simulink model "EcoSIM3_P2_C2_WIP"  (R2014b)
settings: Solver=ode1  SolverMode=SingleTasking  StartTime=0.0  StopTime=inf  FixedStep=0.01  RelTol=1e-3
PostLoadFcn:
  | %, if any(exist('dsrtsu_mdlpostloadfcn', 'file') == [2, 3, 6]), try dsrtsu_mdlpostloadfcn('Execute', bdroot); catch fprintf('Error in PostLoadFcn (dsrtsu_mdlpostloadfcn) for model "%s":\n %s\n', bdroot, lasterr); end, end,
InitFcn:
  | tic
  | %Startup_EcoSIM
values from neighbouring files (symbols this model uses):
  EngPwr = [0 5	10	15	20	25	30	35	40	45	50	55	60	65	70	75	80	85	90	95	100	105	110	115]    [Series_Maps.m]
  EngSpd = [0 477.4645 954.929 1909.858 2864.787 3819.716 4774.645 5729.574 6684.503]    [Series_Maps.m]
  EngTrq = [0	0	0	0	0	0	0	0	0	0	0	0	0	0	0	0	0	0	0	0	0	0	0	0 ... (first row only)    [Series_Maps.m]
  Power = [0 5 10 15 20 25 30]    [Series_Maps.m]
  Torque = [-50,-40,-30,-25,-20,-15,-10,-8,-6,-4,-2,0]    [Series_Maps.m]
undefined symbols (not defined in the file or in its folder): canChannel, Controls, DriveCycles, Driver, EM_EFF_MAP, EM_PwrLoss_MAP, Glbl, Overwritten_Mode, Plants, sigbuilder_block, Trialmap, Veh_Dynamics
libraries: simulink x141, canmsglib x113, fl_lib x104, canlib x89, nesl_utility x56, sdl_lib x29, dspsigops x6, dspswit3 x5, dspstat3 x2, commnoisgen2 x1, dspfdesign x1
(part 5 of 21)

== system EcoSIM3_P2_C2_WIP/Driver/PI Controller/Dyno Data Variant/Coastdown ==
  CycleTime : Constant  Value=Coastdown.time(end)
  From Workspace : FromWorkspace  VariableName=[Coastdown.time',Coastdown.Alpha_percent']  SampleTime=0
  From Workspace1 : FromWorkspace  VariableName=[Coastdown.time',Coastdown.Brake_percent']  SampleTime=0
  From Workspace10 : FromWorkspace  VariableName=[Coastdown.time',Coastdown.bcm_soc']  SampleTime=0
  From Workspace11 : FromWorkspace  VariableName=[Coastdown.time',Coastdown.bcm_cell_tmax']  SampleTime=0
  From Workspace12 : FromWorkspace  VariableName=[Coastdown.time',Coastdown.bcm_cell_tmin']  SampleTime=0
  From Workspace2 : FromWorkspace  VariableName=[Coastdown.time',Coastdown.Speed_m_per_s']  SampleTime=0
  From Workspace3 : FromWorkspace  VariableName=[Coastdown.time',Coastdown.Driver_Req_Trq']  SampleTime=0
  From Workspace4 : FromWorkspace  VariableName=[Coastdown.time',Coastdown.bcm_ibat']  SampleTime=0
  From Workspace5 : FromWorkspace  VariableName=[Coastdown.time',Coastdown.bcm_vbat']  SampleTime=0
  From Workspace6 : FromWorkspace  VariableName=[Coastdown.time',Coastdown.D1_Commanded_Trq']  SampleTime=0
  From Workspace7 : FromWorkspace  VariableName=[Coastdown.time',Coastdown.EM_Trq_Cmd']  SampleTime=0
  From Workspace8 : FromWorkspace  VariableName=[Coastdown.time',Coastdown.Motor_Speed']  SampleTime=0
  From Workspace9 : FromWorkspace  VariableName=[Coastdown.time',Coastdown.D2_Trq_Feedback']  SampleTime=0
  Gain : Gain
  Gain1 : Gain
  Terminator{,1..12} (13 alike) : Terminator
  n : Gain  Gain=-1
  n1 : Gain  Gain=-1
  rpmtoradps : Gain  Gain=-0.1047
  Alpha : Outport
  Beta : Outport  Port=2
  tag scope: CycleTime=global, DynoCellTMax=global, DynoCellTMin=global, DynoSpeed=global
  wires:
  Gain/1 -> Terminator8/1  "Dyno_Brk_Pct"
  From Workspace2/1 -> Terminator/1, [DynoSpeed]  "Dyno_Speed"
  From Workspace/1 -> Gain1/1, Alpha/1
  From Workspace1/1 -> Beta/1, Gain/1
  From Workspace3/1 -> Terminator1/1  "Dyno_Drv_Trq_Req"
  From Workspace5/1 -> Terminator3/1  "Dyno_bcm_vbat"
  From Workspace6/1 -> Terminator4/1  "Dyno_D1_Cmdd_Trq"
  From Workspace7/1 -> Terminator5/1  "Dyno_EM_Trq_Cmd"
  rpmtoradps/1 -> Terminator6/1  "Dyno_MotorSpd_radpers"
  From Workspace8/1 -> rpmtoradps/1  "Dyno_MotorSpd_rpm"
  n/1 -> Terminator7/1  "Dyno_D2_Trq_Fdbk"
  From Workspace9/1 -> n/1
  CycleTime/1 -> [CycleTime]
  From Workspace4/1 -> n1/1
  n1/1 -> Terminator2/1  "Dyno_bcm_ibat"
  From Workspace10/1 -> Terminator9/1  "Dyno_bcm_soc"
  Gain1/1 -> Terminator10/1  "Dyno_Alpha"
  From Workspace11/1 -> [DynoCellTMax], Terminator11/1  "Dyno_bcm_cell_tmax"
  From Workspace12/1 -> [DynoCellTMin], Terminator12/1  "Dyno_bcm_cell_tmin"

== system EcoSIM3_P2_C2_WIP/Driver/PI Controller/Dyno Data Variant/HWFET_150 ==
  CycleTime : Constant  Value=HWFET_150.time(end)
  From Workspace : FromWorkspace  VariableName=[HWFET_150.time',HWFET_150.Alpha_percent']  SampleTime=0
  From Workspace1 : FromWorkspace  VariableName=[HWFET_150.time',HWFET_150.Brake_percent']  SampleTime=0
  From Workspace10 : FromWorkspace  VariableName=[HWFET_150.time',HWFET_150.bcm_soc']  SampleTime=0
  From Workspace11 : FromWorkspace  VariableName=[HWFET_150.time',HWFET_150.bcm_cell_tmax']  SampleTime=0
  From Workspace12 : FromWorkspace  VariableName=[HWFET_150.time',HWFET_150.bcm_cell_tmin']  SampleTime=0
  From Workspace2 : FromWorkspace  VariableName=[HWFET_150.time',HWFET_150.Speed_m_per_s']  SampleTime=0
  From Workspace3 : FromWorkspace  VariableName=[HWFET_150.time',HWFET_150.Driver_Req_Trq']  SampleTime=0
  From Workspace4 : FromWorkspace  VariableName=[HWFET_150.time',HWFET_150.bcm_ibat']  SampleTime=0
  From Workspace5 : FromWorkspace  VariableName=[HWFET_150.time',HWFET_150.bcm_vbat']  SampleTime=0
  From Workspace6 : FromWorkspace  VariableName=[HWFET_150.time',HWFET_150.D1_Commanded_Trq']  SampleTime=0
  From Workspace7 : FromWorkspace  VariableName=[HWFET_150.time',HWFET_150.EM_Trq_Cmd']  SampleTime=0
  From Workspace8 : FromWorkspace  VariableName=[HWFET_150.time',HWFET_150.Motor_Speed']  SampleTime=0
  From Workspace9 : FromWorkspace  VariableName=[HWFET_150.time',HWFET_150.D2_Trq_Feedback']  SampleTime=0
  Gain : Gain
  Gain1 : Gain
  Terminator{,1..12} (13 alike) : Terminator
  Transfer Fcn : TransferFcn  Denominator=[1 1]
  n : Gain  Gain=-1
  n1 : Gain  Gain=-1
  rpmtoradps : Gain  Gain=-0.1047
  Alpha : Outport
  Beta : Outport  Port=2
  tag scope: CycleTime=global, DynoCellTMax=global, DynoCellTMin=global, DynoSpeed=global
  wires:
  Transfer Fcn/1 -> Terminator/1, [DynoSpeed]  "Dyno_Speed"
  Gain1/1 -> Terminator10/1  "Dyno_Alpha"
  From Workspace10/1 -> Terminator9/1  "Dyno_bcm_soc"
  n1/1 -> Terminator2/1  "Dyno_bcm_ibat"
  From Workspace4/1 -> n1/1
  Gain/1 -> Terminator8/1  "Dyno_Brk_Pct"
  From Workspace2/1 -> Transfer Fcn/1
  From Workspace/1 -> Alpha/1, Gain1/1
  From Workspace1/1 -> Beta/1, Gain/1
  From Workspace3/1 -> Terminator1/1  "Dyno_Drv_Trq_Req"
  From Workspace5/1 -> Terminator3/1  "Dyno_bcm_vbat"
  From Workspace6/1 -> Terminator4/1  "Dyno_D1_Cmdd_Trq"
  From Workspace7/1 -> Terminator5/1  "Dyno_EM_Trq_Cmd"
  rpmtoradps/1 -> Terminator6/1  "Dyno_MotorSpd_radpers"
  From Workspace8/1 -> rpmtoradps/1  "Dyno_MotorSpd_rpm"
  n/1 -> Terminator7/1  "Dyno_D2_Trq_Fdbk"
  From Workspace9/1 -> n/1
  CycleTime/1 -> [CycleTime]
  From Workspace11/1 -> [DynoCellTMax], Terminator11/1  "Dyno_bcm_cell_tmax"
  From Workspace12/1 -> [DynoCellTMin], Terminator12/1  "Dyno_bcm_cell_tmin"

== system EcoSIM3_P2_C2_WIP/Driver/PI Controller/Dyno Data Variant/US06_150 ==
  CycleTime : Constant  Value=US06_150.time(end)
  From Workspace : FromWorkspace  VariableName=[US06_150.time',US06_150.Alpha_percent']  SampleTime=0
  From Workspace1 : FromWorkspace  VariableName=[US06_150.time',US06_150.Brake_percent']  SampleTime=0
  From Workspace10 : FromWorkspace  VariableName=[US06_150.time',US06_150.bcm_soc']  SampleTime=0
  From Workspace11 : FromWorkspace  VariableName=[US06_150.time',US06_150.bcm_cell_tmax']  SampleTime=0
  From Workspace12 : FromWorkspace  VariableName=[US06_150.time',US06_150.bcm_cell_tmin']  SampleTime=0
  From Workspace2 : FromWorkspace  VariableName=[US06_150.time',US06_150.Speed_m_per_s']  SampleTime=0
  From Workspace3 : FromWorkspace  VariableName=[US06_150.time',US06_150.Driver_Req_Trq']  SampleTime=0
  From Workspace4 : FromWorkspace  VariableName=[US06_150.time',US06_150.bcm_ibat']  SampleTime=0
  From Workspace5 : FromWorkspace  VariableName=[US06_150.time',US06_150.bcm_vbat']  SampleTime=0
  From Workspace6 : FromWorkspace  VariableName=[US06_150.time',US06_150.D1_Commanded_Trq']  SampleTime=0
  From Workspace7 : FromWorkspace  VariableName=[US06_150.time',US06_150.EM_Trq_Cmd']  SampleTime=0
  From Workspace8 : FromWorkspace  VariableName=[US06_150.time',US06_150.Motor_Speed']  SampleTime=0
  From Workspace9 : FromWorkspace  VariableName=[US06_150.time',US06_150.D2_Trq_Feedback']  SampleTime=0
  Gain : Gain
  Gain1 : Gain
  Terminator{,1..12} (13 alike) : Terminator
  Transfer Fcn : TransferFcn  Denominator=[1 1]
  n : Gain  Gain=-1
  n1 : Gain  Gain=-1
  rpmtoradps : Gain  Gain=-0.1047
  Alpha : Outport
  Beta : Outport  Port=2
  tag scope: CycleTime=global, DynoCellTMax=global, DynoCellTMin=global, DynoSpeed=global
  wires:
  CycleTime/1 -> [CycleTime]
  From Workspace9/1 -> n/1
  n/1 -> Terminator7/1  "Dyno_D2_Trq_Fdbk"
  From Workspace8/1 -> rpmtoradps/1  "Dyno_MotorSpd_rpm"
  rpmtoradps/1 -> Terminator6/1  "Dyno_MotorSpd_radpers"
  From Workspace7/1 -> Terminator5/1  "Dyno_EM_Trq_Cmd"
  From Workspace6/1 -> Terminator4/1  "Dyno_D1_Cmdd_Trq"
  From Workspace5/1 -> Terminator3/1  "Dyno_bcm_vbat"
  From Workspace3/1 -> Terminator1/1  "Dyno_Drv_Trq_Req"
  From Workspace1/1 -> Gain/1, Beta/1
  From Workspace/1 -> Gain1/1, Alpha/1
  From Workspace2/1 -> Transfer Fcn/1
  Gain/1 -> Terminator8/1  "Dyno_Brk_Pct"
  From Workspace4/1 -> n1/1
  n1/1 -> Terminator2/1  "Dyno_bcm_ibat"
  From Workspace10/1 -> Terminator9/1  "Dyno_bcm_soc"
  Gain1/1 -> Terminator10/1  "Dyno_Alpha"
  Transfer Fcn/1 -> [DynoSpeed], Terminator/1  "Dyno_Speed"
  From Workspace11/1 -> [DynoCellTMax], Terminator11/1  "Dyno_bcm_cell_tmax"
  From Workspace12/1 -> [DynoCellTMin], Terminator12/1  "Dyno_bcm_cell_tmin"

== system EcoSIM3_P2_C2_WIP/GCM/GCM_IO/VNT Kvaser/CAN Rx ==
  note: This is a digital signal. So use from goto.
  Ground : Ground
  CAN : Outport
  wires:
  Ground/1 -> CAN/1

== system EcoSIM3_P2_C2_WIP/GCM/GCM_IO/VNT Kvaser/CAN Tx ==
  CAN : Inport
  Bus Selector : BusSelector  OutputSignals=charge_mode_request
  CAN Pack6 : canmsglib/CAN Pack  CANdbFile=C:\Users\EcoCAR_HIL\Documents\Khanna\EcoSIM3_P1_0_PHEV_TCU\Final_DBC\EcoCAR3_Controls_Development.dbc  MsgList=GCM_Transmit_MSG096  MsgName=GCM_Transmit_MSG096  MsgIDType=Standard (11-bit identifier)  MsgIdentifier=96  MsgLength=1  SignalInfo=charge_mode_request$7$1$2$2$1$0$1$0$0$1$#  NSignals=1  StartBits=str2num('[int32(7)]')  SignalSizes=str2num('[int32(1)]')  ByteOrders=str2num('[int32(2)]')  DataTypes=str2num('[int32(2)]')  MultiplexTypes=str2num('[int32(1)]')  MultiplexValues=str2num('[double(0)]')  Factors=str2num('[double(1)]')  Offsets=str2num('[double(0)]')  Minimums=str2num('[double(0)]')  Maximums=str2num('[double(1)]')  Remote=off
      settings: DataFormat=CANdb specified signals
  CAN Transmit6 : canlib/CAN Transmit  BlockHandle=888.0005  DeviceMenu=(none)  Device=Kvaser Virtual 1 (Channel 1)  ObjConstructor=canChannel('Kvaser', 'Virtual 1', 1)  EnablePeriodicTransmit=off  MessagePeriod=1.000
  Rate Transition : RateTransition
  wires:
  CAN Pack6/1 -> CAN Transmit6/1
  CAN/1 -> Bus Selector/1
  Bus Selector/1 -> Rate Transition/1  "<charge_mode_request>"
  Rate Transition/1 -> CAN Pack6/1

== system EcoSIM3_P2_C2_WIP/GCM/GCM_IO/VNT Kvaser/Electrical Rx ==
  Bus Creator{,1..3} (4 alike) : BusCreator  Inputs=1
  Bus Creator5 : BusCreator  Inputs=2
  Bus Selector : BusSelector  OutputSignals=GM_Electrical_Out.Key_State,Brusa_Electrical_Out.GCM_Wakeup_charge
  Electrical : Outport
  wires:
  [VNT_Electrical_From_SoftECU] -> Bus Selector/1
  Bus Creator5/1 -> Electrical/1
  Bus Creator3/1 -> Bus Creator5/2  "Brusa_Transmit"
  Bus Creator1/1 -> Bus Creator5/1  "GM_Transmit"
  Bus Creator2/1 -> Bus Creator3/1  "Brusa_Electrical_Out"
  Bus Creator/1 -> Bus Creator1/1  "GM_Electrical_Out"
  Bus Selector/1 -> Bus Creator/1  "<Key_State>"
  Bus Selector/2 -> Bus Creator2/1  "<GCM_Wakeup_charge>"

== system EcoSIM3_P2_C2_WIP/GCM/GCM_IO/VNT Kvaser/Electrical Tx ==
  Electrical : Inport
  tag scope: VNT_Electrical_FromGCM=global
  wires:
  Electrical/1 -> [VNT_Electrical_FromGCM]

== system EcoSIM3_P2_C2_WIP/GCM/GCM_IO/VNT Kvaser/Spine ==
  note: This is a digital signal. So use from goto.
  Electrical Rx : Inport
  CAN Rx : Inport  Port=2
  Bus Selector : BusSelector  OutputSignals=GCM_Electrical_Out,GCM_CAN_Out
  Terminator : Terminator
  Electrical Tx : Outport
  CAN Tx : Outport  Port=2
  tag scope: GCM_from_CAN=global
  wires:
  [GCM_To_CAN] -> Bus Selector/1
  Electrical Rx/1 -> [GCM_from_CAN]
  CAN Rx/1 -> Terminator/1
  Bus Selector/1 -> Electrical Tx/1  "<GCM_Electrical_Out>"
  Bus Selector/2 -> CAN Tx/1  "<GCM_CAN_Out>"

== system EcoSIM3_P2_C2_WIP/GCM/GCM_IO/VNT Vector/CAN Rx ==
  note: This is a digital signal. So use from goto.
  Bus Creator : BusCreator  Inputs=2
  CAN Receive : canlib/CAN Receive  BlockHandle=937.0007  DeviceMenu=(none)  Device=Vector Virtual 1 (Channel 1)  ObjConstructor=canChannel('Vector', 'Virtual 1', 1)  EnableStandardIDsFilter=off  StandardIDs=95  EnableExtendedIDsFilter=off  ExtendedIDs=0  SampleTime=0.01  MsgsPerTimestep=1  StdIDsCombo=Allow only  ExtIDsCombo=Allow all  InternalFilterUpdateStatus=on
  CAN Unpack : canmsglib/CAN Unpack  CANdbFile=C:\Box Sync\EcoCAR 3\SMS\EcoSIM3_P2_C2\MIL\Final_DBC\EcoCAR3_Controls_Development.dbc  MsgList=GCM_Receive_MSG095  MsgName=GCM_Receive_MSG095  MsgIDType=Standard (11-bit identifier)  MsgIdentifier=95  MsgLength=2  SignalInfo=BAS_Relay_Close$7$1$2$2$1$0$1$0$0$1$#BCM_Relay_Close$6$1$2$2$1$0$1$0$0$1$#Clutch_Status$14$2$2$2$1$0$1$0$0$3$#ECM_Relay_Close$5$1$2$2$1$0$1$0$0$1$#EM_Relay_Close$4$1$2$2$1$0$1$0$0$1$#GCM_Gear_Request$1$3$2$1$1$0$1$3$-1$6$#  NSignals=6  IDPort=off  TimestampPort=off  ErrorPort=off  RemotePort=off  LengthPort=off  StatusPort=off  StartBits=str2num('[int32(7);int32(6);int32(14);int32(5);int32(4);int32(1)]')  SignalSizes=str2num('[int32(1);int32(1);int32(2);int32(1);int32(1);int32(3)]')  ByteOrders=str2num('[int32(2);int32(2);int32(2);int32(2);int32(2);int32(2)]')  DataTypes=str2num('[int32(2);int32(2);int32(2);int32(2);int32(2);int32(1)]')  MultiplexTypes=str2num('[int32(1);int32(1);int32(1);int32(1);int32(1);int32(1)]')  MultiplexValues=str2num('[double(0);double(0);double(0);double(0);double(0);double(0)]')  Factors=str2num('[double(1);double(1);double(1);double(1);double(1);double(1)]')  Offsets=str2num('[double(0);double(0);double(0);double(0);double(0);double(3)]')  Minimums=str2num('[double(0);double(0);double(0);double(0);double(0);double(-1)]')  Maximums=str2num('[double(1);double(1);double(3);double(1);double(1);double(6)]')
      settings: DataFormat=CANdb specified signals
  Scope : Scope
      settings: SaveName=ScopeData63
  Terminator : Terminator
  CAN : Outport
  wires:
  CAN Receive/2 -> CAN Unpack/1
  CAN Receive/1 -> Terminator/1
  CAN Unpack/3 -> Bus Creator/1  "Clutch_Status"
  CAN Unpack/6 -> Scope/1, Bus Creator/2  "GCM_Gear_Request"
  Bus Creator/1 -> CAN/1  "GCM_Messages_Transmission"

== system EcoSIM3_P2_C2_WIP/GCM/GCM_IO/VNT Vector/CAN Tx ==
  CAN : Inport
  Bus Selector : BusSelector  OutputSignals=Shift_Status_to_MABx.GCM_Reported_Gear,Shift_Status_to_MABx.Shift_Complete,charge_mode_request
  CAN Pack6 : canmsglib/CAN Pack  CANdbFile=C:\Box Sync\EcoCAR 3\SMS\EcoSIM3_P2_C2\MIL\Final_DBC\EcoCAR3_Controls_Development.dbc  MsgList=GCM_Transmit_MSG052  MsgName=GCM_Transmit_MSG052  MsgIDType=Standard (11-bit identifier)  MsgIdentifier=52  MsgLength=2  SignalInfo=GCM_Heartbeat$2$5$2$2$1$0$1$0$0$31$#GCM_Reported_Gear$13$3$2$1$1$0$1$3$-1$6$#Shift_Complete$1$1$2$2$1$0$1$0$0$1$#charge_mode_request$7$1$2$2$1$0$1$0$0$1$#  NSignals=4  StartBits=str2num('[int32(2);int32(13);int32(1);int32(7)]')  SignalSizes=str2num('[int32(5);int32(3);int32(1);int32(1)]')  ByteOrders=str2num('[int32(2);int32(2);int32(2);int32(2)]')  DataTypes=str2num('[int32(2);int32(1);int32(2);int32(2)]')  MultiplexTypes=str2num('[int32(1);int32(1);int32(1);int32(1)]')  MultiplexValues=str2num('[double(0);double(0);double(0);double(0)]')  Factors=str2num('[double(1);double(1);double(1);double(1)]')  Offsets=str2num('[double(0);double(3);double(0);double(0)]')  Minimums=str2num('[double(0);double(-1);double(0);double(0)]')  Maximums=str2num('[double(31);double(6);double(1);double(1)]')  Remote=off
      settings: DataFormat=CANdb specified signals
  CAN Transmit6 : canlib/CAN Transmit  BlockHandle=954.0005  DeviceMenu=(none)  Device=Vector Virtual 1 (Channel 1)  ObjConstructor=canChannel('Vector', 'Virtual 1', 1)  EnablePeriodicTransmit=off  MessagePeriod=1.000
  Rate Transition : RateTransition
  Rate Transition1 : RateTransition
  Rate Transition2 : RateTransition
  wires:
  CAN Pack6/1 -> CAN Transmit6/1
  CAN/1 -> Bus Selector/1
  Bus Selector/3 -> Rate Transition/1  "<charge_mode_request>"
  Rate Transition/1 -> CAN Pack6/4
  Bus Selector/2 -> Rate Transition1/1  "<Shift_Complete>"
  Rate Transition1/1 -> CAN Pack6/3
  Bus Selector/1 -> Rate Transition2/1  "<GCM_Reported_Gear>"
  Rate Transition2/1 -> CAN Pack6/2

== system EcoSIM3_P2_C2_WIP/GCM/GCM_IO/VNT Vector/Electrical Rx ==
  Bus Creator{,1..4} (5 alike) : BusCreator  Inputs=1
  Bus Creator5 : BusCreator  Inputs=3
  Bus Selector : BusSelector  OutputSignals=GM_Electrical_Out.Accessory_Wake,Brusa_Electrical_Out.GCM_Wakeup_charge,Mastershift_Electrical_Out
  Electrical : Outport
  wires:
  [VNT_Electrical_From_SoftECU] -> Bus Selector/1
  Bus Creator5/1 -> Electrical/1
  Bus Creator3/1 -> Bus Creator5/2  "Brusa_Transmit"
  Bus Creator1/1 -> Bus Creator5/1  "GM_Transmit"
  Bus Creator2/1 -> Bus Creator3/1  "Brusa_Electrical_Out"
  Bus Creator/1 -> Bus Creator1/1  "GM_Electrical_Out"
  Bus Selector/1 -> Bus Creator/1  "<Accessory_Wake>"
  Bus Selector/2 -> Bus Creator2/1  "<GCM_Wakeup_charge>"
  Bus Creator4/1 -> Bus Creator5/3  "Mastershift_Transmit"
  Bus Selector/3 -> Bus Creator4/1  "<Mastershift_Electrical_Out>"

== system EcoSIM3_P2_C2_WIP/GCM/GCM_IO/VNT Vector/Electrical Tx ==
  Electrical : Inport
  tag scope: VNT_Electrical_FromGCM=global
  wires:
  Electrical/1 -> [VNT_Electrical_FromGCM]

== system EcoSIM3_P2_C2_WIP/GCM/GCM_IO/VNT Vector/Spine ==
  note: This is a digital signal. So use from goto.
  Electrical Rx : Inport
  CAN Rx : Inport  Port=2
  Bus Creator : BusCreator
  Bus Selector : BusSelector  OutputSignals=GCM_Electrical_Out,GCM_CAN_Out
  Bus Selector1 : BusSelector  OutputSignals=GM_Transmit,Brusa_Transmit,Mastershift_Transmit
  Electrical Tx : Outport
  CAN Tx : Outport  Port=2
  tag scope: GCM_from_CAN=global
  wires:
  [GCM_To_CAN] -> Bus Selector/1
  Bus Selector/1 -> Electrical Tx/1  "<GCM_Electrical_Out>"
  Bus Selector/2 -> CAN Tx/1  "<GCM_CAN_Out>"
  Electrical Rx/1 -> Bus Selector1/1
  Bus Selector1/3 -> Bus Creator/3  "<Mastershift_Transmit>"
  Bus Selector1/1 -> Bus Creator/1  "<GM_Transmit>"
  Bus Selector1/2 -> Bus Creator/2  "<Brusa_Transmit>"
  CAN Rx/1 -> Bus Creator/4
  Bus Creator/1 -> [GCM_from_CAN]

== system EcoSIM3_P2_C2_WIP/Powertrain/Accessories Power Module/CAN_Receive/Signal Builder ==
  Demux : Demux  Tag=STV Demux  Outputs=3
  FromWs : FromWorkspace  Tag=STV FromWs  VariableName=tuvar  SampleTime=0
      SigBuilderData=|
      | common.afterFinalStr = 'Extrapolate'
      | common.sampleTime = 0
      | dataSet.timeRange = [0 10]
      | dataSet.name = 'Group 1'
      | sbobj.Groups.Name = 'Group 1'
      | sbobj.Groups.Signals(1).Name = 'Signal 1'
      | sbobj.Groups.Signals(1).XData = [0 2 2 4 4 7 10]
      | sbobj.Groups.Signals(1).YData = [0 0 1 1 0 1 6]
      | sbobj.Groups.Signals(2).Name = 'Signal 2'
      | sbobj.Groups.Signals(2).XData = [0 4 5 7 10]
      | sbobj.Groups.Signals(2).YData = [0 0 1 0 1]
      | sbobj.Groups.Signals(3).Name = 'Signal 4'
      | sbobj.Groups.Signals(3).XData = [0 4 4 10]
      | sbobj.Groups.Signals(3).YData = [0 0 1 1]
  Signal 1 : Outport  Tag=STV Outport
  Signal 2 : Outport  Tag=STV Outport  Port=2
  Signal 4 : Outport  Tag=STV Outport  Port=3
  wires:
  Demux/1 -> Signal 1/1
  FromWs/1 -> Demux/1
  Demux/2 -> Signal 2/1
  Demux/3 -> Signal 4/1

== system EcoSIM3_P2_C2_WIP/Powertrain/Accessories Power Module/Component Power/HVAC ==
  AC_Mode : Inport
  AC_Press_bar : Inport  Port=2
  AC_Engagement_pressure : Inport  Port=3
  AC_max_pressure : Inport  Port=4
  Current : Inport  Port=5
  Voltage : Inport  Port=6
  HVAC softECU : Stateflow chart  TreatAsAtomicUnit=on
  Product : Product  Inputs=3
  HVAC Pwr_W : Outport
  wires:
  AC_Mode/1 -> HVAC softECU/1(AC_Mode)
  AC_Press_bar/1 -> HVAC softECU/2(AC_Press_bar)
  AC_Engagement_pressure/1 -> HVAC softECU/3(AC_engagement_pressure)
  AC_max_pressure/1 -> HVAC softECU/4(AC_max_pressure)
  HVAC softECU/1(Compressor_status) -> Product/1
  Voltage/1 -> Product/2
  Current/1 -> Product/3
  Product/1 -> HVAC Pwr_W/1

== system EcoSIM3_P2_C2_WIP/Powertrain/Accessories Power Module/Component Power/Parameters ==
  note: Parameter Order:
      | 1) Update Rate
      | 2) Scale Error
      | 3) Bias Error
      | 4) Noise Amplitude
      | 5) Latency
      | 6) Quantization
      | 7) Filter Tau
  BiasError : Constant  Value=0
  Bus Creator : BusCreator  Inputs=8
  Enable : Constant
  FilterTau : Constant
  Latency : Constant  Value=0.09
  NoiseAmplitude : Constant  Value=0.1034
  Quantization : Constant  Value=0.1
  ScaleError : Constant
  UpdateRate : Constant
  P : Outport
  wires:
  Bus Creator/1 -> P/1
  Enable/1 -> Bus Creator/8  "Enable_Corrupter"
  Quantization/1 -> Bus Creator/6  "Quantization"
  Latency/1 -> Bus Creator/5  "Latency"
  FilterTau/1 -> Bus Creator/7  "Filter_Tau"
  NoiseAmplitude/1 -> Bus Creator/4  "Noise_Amplitude"
  BiasError/1 -> Bus Creator/3  "Bias_Error"
  ScaleError/1 -> Bus Creator/2  "Scale_Error"
  UpdateRate/1 -> Bus Creator/1  "Update_Rate"

== system EcoSIM3_P2_C2_WIP/Powertrain/Accessories Power Module/Component Power/The Corrupter ==
  note: Parameter Values-
      | Update Rate - 1
      | Scale Error - 1
      | Bias Error - 2
      | Noise Amplitude - 3.716
      | Latency - 0.09
      | Quantization - 0.5
      | Filter Tau - 1
      | Enable - 1
  note: Rate 1 = .01 sec
      | Rate 2 = .03 sec
      | Rate 3 = .02 sec
  note: Order of Operations:
      | 1) Scale Error
      | 2) Bias Error
      | 3) Low pass filter
      | 4) Noise
      | 5) Quantization
      | 6) Latency
      | 7) Sample and hold
  note: Parameter Order:
      | 1) Update Rate
      | 2) Scale Error
      | 3) Bias Error
      | 4) Noise Amplitude
      | 5) Latency
      | 6) Quantization
      | 7) Filter Tau
      | 8) Corruption Enable
  Signal In : Inport
  Noise Parameters : Inport  Port=2
  Abs : Abs
  Bus Selector : BusSelector  OutputSignals=Update_Rate,Scale_Error,Bias_Error,Noise_Amplitude,Latency,Quantization,Filter_Tau,Enable_Corrupter
  Compare To Constant : simulink/Logic and Bit Operations/Compare To Constant  relop=~=  const=0  OutDataTypeStr=boolean
  Enabled Subsystem : Subsystem  TreatAsAtomicUnit=on
  From : From  Commented=on  GotoTag=Rate_1
  From1 : From  Commented=on  GotoTag=Rate_2
  From2 : From  Commented=on  GotoTag=Rate_3
  Gaussian Noise Generator : commnoisgen2/Gaussian Noise Generator  m=0  d=1  s=41  Ts=0.1  frameBased=off  sampPerFrame=1  orient=off  outDataType=double
  "Latency " : VariableTransportDelay  MaximumPoints=2048  ZeroDelay=on
  Memory1 : Memory
  Multiport Switch : MultiPortSwitch  Inputs=4
  Multiport Switch1 : MultiPortSwitch  Inputs=2
  One : Constant
  One1 : Constant  Value=4
  One2 : Constant  Value=0.01
  One3 : Constant  Value=0.03
  One4 : Constant  Value=0.02
  Product{,1..2,5} (4 alike) : Product  RndMeth=Zero
  Product3 : Product  Inputs=*/  RndMeth=Zero
  Product4 : Product  Inputs=*/  RndMeth=Zero
  Rounding Function : Rounding  Operator=round
  Rounding Function1 : Rounding  Operator=round
  Saturation : Saturate  UpperLimit=inf  LowerLimit=.0001
  Saturation1 : Saturate  UpperLimit=inf  LowerLimit=0
  Saturation2 : Saturate  UpperLimit=1  LowerLimit=0
  Saturation3 : Saturate  UpperLimit=3  LowerLimit=1
  Saturation4 : Saturate  UpperLimit=2  LowerLimit=1
  Sum : Sum  Inputs=|++
  Sum1 : Sum  Inputs=|++
  Sum2 : Sum  Inputs=|+-
  Switch Logic : Subsystem
  Switch Logic1 : Subsystem
  Transmit Rate and/or Sample Rate : dspsigops/Sample and Hold  trig=Rising edge  initCond=0  latchinput=off
  Signal Out : Outport
  wires:
  Memory1/1 -> Sum2/2
  Switch Logic1/1(Out1) -> Sum/1
  Compare To Constant/1 -> Enabled Subsystem/Enable
  Signal In/1 -> Product5/1, Product1/1, Switch Logic/1(NonCorrupted)
  Switch Logic/1(Signal Out) -> Signal Out/1
  Multiport Switch1/1 -> Switch Logic/2(Corrupted)
  Saturation4/1 -> Multiport Switch1/1
  Product3/1 -> "Latency "/1
  Product/1 -> Sum/2
  Gaussian Noise Generator/1 -> Product/1
  Enabled Subsystem/1(Out1) -> Memory1/1, Switch Logic1/1(F)
  "Latency "/1 -> Multiport Switch1/2, Transmit Rate and/or Sample Rate/1
  Transmit Rate and/or Sample Rate/1 -> Multiport Switch1/3
  Product1/1 -> Sum1/1
  Product2/1 -> Rounding Function/1
  Rounding Function/1 -> Product3/1
  Product4/1 -> Product2/2, Product3/2
  Sum/1 -> Product2/1
  One/1 -> Product4/1
  Multiport Switch/1 -> Transmit Rate and/or Sample Rate/Trigger
  Sum2/1 -> Enabled Subsystem/1(In1)
  Sum1/1 -> Switch Logic1/3(NF), Sum2/1
  One3/1 -> Multiport Switch/3
  One4/1 -> Multiport Switch/4
  One2/1 -> Multiport Switch/2
  Bus Selector/1 -> Saturation3/1  "<Update_Rate>"
  Abs/1 -> Saturation1/1
  Saturation/1 -> Product4/2
  Saturation1/1 -> Product/2
  Saturation2/1 -> "Latency "/2
  Saturation3/1 -> Rounding Function1/1
  Rounding Function1/1 -> Saturation4/1, Multiport Switch/1
  One1/1 -> Multiport Switch/5
  Noise Parameters/1 -> Bus Selector/1
  Bus Selector/2 -> Product1/2  "<Scale_Error>"
  Bus Selector/3 -> Sum1/2  "<Bias_Error>"
  Bus Selector/4 -> Product5/2  "<Noise_Amplitude>"
  Bus Selector/5 -> Saturation2/1  "<Latency>"
  Bus Selector/6 -> Saturation/1  "<Quantization>"
  Bus Selector/7 -> Enabled Subsystem/2(In2), Compare To Constant/1  "<Filter_Tau>"
  Bus Selector/8 -> Switch Logic/3(Logic)  "<Enable_Corrupter>"
  Product5/1 -> Abs/1

== system EcoSIM3_P2_C2_WIP/Powertrain/Accessories Power Module/Subsystem/Algorithm ==
  Inputs : Inport
  Bus Creator : BusCreator  Inputs=13
  Bus Selector : BusSelector  OutputSignals=DCDC_SoftECU_Receive.DCDC_Electrical.DCDC_Powerup,DCDC_SoftECU_Receive.DCDC_CAN.PTEI_Hybrid_General_Status_1.LowVoltEnblRq,ESS_Transmit.ESS_CAN_Out.BCM_Status.bcm_mainc_stat,DCDC_SoftECU_Receive.DCDC_CAN.PTEI_Hybrid_General_Status_1.LwVltStpntCmnd,APM_Sensor_Out.Temperature_Sensors.Fault,ESS_Transmit.ESS_CAN_Out.BCM_Status.bcm_vbat,Accessories_Power_In_W,APM_Sensor_Out.Temperature_Sensors.AccPwrModTmp1,APM_Sensor_Out.Temperature_Sensors.AccPwrModTmp2,APM_Sensor_Out.Electrical_Sensors.APMLwVltOtptCrntUns,APM_Sensor_Out.Electrical_Sensors.AccPwrMdlHiVltInpCrnt
  CAN fault : Stateflow chart  TreatAsAtomicUnit=on
  Constant{,1..4} (5 alike) : Constant  Value=0  OutDataTypeStr=boolean
  DC-DC SoftECU : Stateflow chart  TreatAsAtomicUnit=on
  Data Type Conversion1 : DataTypeConversion  OutDataTypeStr=boolean
  Scope : Scope
  Scope1 : Scope
  Scope2 : Scope
      settings: YMin=-10  YMax=10  SaveName=ScopeData4
  Outputs : Outport
  wires:
  DC-DC SoftECU/1(State) -> Scope1/1
  CAN fault/1(CANdown) -> DC-DC SoftECU/1(CANdown)
  Inputs/1 -> Bus Selector/1
  DC-DC SoftECU/2(AccPwrMdlLowVlt) -> Scope2/1, Bus Creator/1
  DC-DC SoftECU/3(AccPwrMdlLwVltSysFld) -> Data Type Conversion1/1
  Bus Creator/1 -> Outputs/1  "APM_SoftECU_Out"
  CAN fault/2(state) -> Scope/1
  Bus Selector/1 -> DC-DC SoftECU/2(PowerUp), CAN fault/1(PowerUp)  "<DCDC_Powerup>"
  Bus Selector/2 -> CAN fault/2(LowVoltEnblRq), DC-DC SoftECU/3(LowVoltEnblRq)  "<LowVoltEnblRq>"
  Bus Selector/3 -> DC-DC SoftECU/4(bcm_mainc_stat)  "<bcm_mainc_stat>"
  Bus Selector/4 -> DC-DC SoftECU/5(LwVltStpntCmnd)  "<LwVltStpntCmnd>"
  Data Type Conversion1/1 -> Bus Creator/2  "AccPwrMdlLwVltSysFld"
  Bus Selector/11 -> Bus Creator/8  "<AccPwrMdlHiVltInpCrnt>"
  Bus Selector/10 -> Bus Creator/7  "<APMLwVltOtptCrntUns>"
  Bus Selector/9 -> Bus Creator/6  "<AccPwrModTmp2>"
  Bus Selector/8 -> Bus Creator/5  "<AccPwrModTmp1>"
  Constant/1 -> Bus Creator/9  "AccPwrMdlHiVltInpCrntV"
  Constant1/1 -> Bus Creator/10  "AccPwrMdlLowVltV"
  Constant2/1 -> Bus Creator/11  "AccPwrModTmp1V"
  Constant3/1 -> Bus Creator/12  "AccPwrModTmp2V"
  Constant4/1 -> Bus Creator/13  "APMLwVltOtptCrntUnsV"
  Bus Selector/5 -> DC-DC SoftECU/6(Fault)  "<Fault>"
  Bus Selector/6 -> DC-DC SoftECU/7(bcmVbat), Bus Creator/3  "<bcm_vbat>"
  Bus Selector/7 -> DC-DC SoftECU/8(PowerReq), Bus Creator/4  "<Accessories_Power_In_W>"

== system EcoSIM3_P2_C2_WIP/Powertrain/Accessories Power Module/Subsystem/Inputs ==
  CAN_In : Inport
  Sensors : Inport  Port=2
  Bus Creator : BusCreator
  Bus Selector2 : BusSelector  OutputSignals=DCDC_SoftECU_Receive,ESS_Transmit
  Bus Selector3 : BusSelector  OutputSignals=Accessories_Power_In_W,APM_Sensor_Out
  To_Algorithm : Outport
  wires:
  Sensors/1 -> Bus Selector3/1
  CAN_In/1 -> Bus Selector2/1
  Bus Selector2/1 -> Bus Creator/1  "<DCDC_SoftECU_Receive>"
  Bus Selector2/2 -> Bus Creator/2  "<ESS_Transmit>"
  Bus Creator/1 -> To_Algorithm/1
  Bus Selector3/1 -> Bus Creator/3  "<Accessories_Power_In_W>"
  Bus Selector3/2 -> Bus Creator/4  "<APM_Sensor_Out>"

== system EcoSIM3_P2_C2_WIP/Powertrain/Accessories Power Module/Subsystem/Outputs ==
  From Algorithm : Inport
  Bus Creator : BusCreator  Inputs=11
  Bus Creator1 : BusCreator  Inputs=1
  Bus Creator2 : BusCreator  Inputs=3
  Bus Selector : BusSelector  OutputSignals=AccPwrMdlHiVltInpCrntV,AccPwrMdlLowVltV,AccPwrModTmp1V,AccPwrModTmp2V,APMLwVltOtptCrntUnsV,APMLwVltOtptCrntUns,AccPwrMdlHiVltInpCrnt,AccPwrMdlLwVltSysFld,AccPwrModTmp1,AccPwrModTmp2,AccPwrMdlLowVlt,Accessories_Power_In_W,bcm_vbat
  To ECU : Outport
  Actuator_Cmds : Outport  Port=2
  wires:
  Bus Creator/1 -> Bus Creator1/1  "Accessory_Pwr_Mod_Gen_Status_1"
  From Algorithm/1 -> Bus Selector/1
  Bus Selector/11 -> Bus Creator2/1, Bus Creator/11  "<AccPwrMdlLowVlt>"
  Bus Selector/6 -> Bus Creator/6  "<APMLwVltOtptCrntUns>"
  Bus Selector/8 -> Bus Creator/8  "<AccPwrMdlLwVltSysFld>"
  Bus Selector/9 -> Bus Creator/9  "<AccPwrModTmp1>"
  Bus Selector/10 -> Bus Creator/10  "<AccPwrModTmp2>"
  Bus Selector/7 -> Bus Creator/7  "<AccPwrMdlHiVltInpCrnt>"
  Bus Creator1/1 -> To ECU/1  "APM_CAN_Out"
  Bus Creator2/1 -> Actuator_Cmds/1  "APM_Actuator_Out"
  Bus Selector/12 -> Bus Creator2/2  "<Accessories_Power_In_W>"
  Bus Selector/13 -> Bus Creator2/3  "<bcm_vbat>"
  Bus Selector/1 -> Bus Creator/1  "<AccPwrMdlHiVltInpCrntV>"
  Bus Selector/2 -> Bus Creator/2  "<AccPwrMdlLowVltV>"
  Bus Selector/3 -> Bus Creator/3  "<AccPwrModTmp1V>"
  Bus Selector/4 -> Bus Creator/4  "<AccPwrModTmp2V>"
  Bus Selector/5 -> Bus Creator/5  "<APMLwVltOtptCrntUnsV>"

== system EcoSIM3_P2_C2_WIP/Powertrain/BAS Motor/ Compnent Model/Actuators ==
  note: Actuator Model or a Signal Pass-through, Remove the bus if you are passing through all the signals
  ActuatorInputs : Inport
  Actuator Outputs : Outport
  wires:
  ActuatorInputs/1 -> Actuator Outputs/1

== system EcoSIM3_P2_C2_WIP/Powertrain/BAS Motor/ Compnent Model/Plant ==
  note: Component Level Performance Maps
  note: Three kinds of Outputs:
      | 1.To_sensors: Signals that can actually be sensed through Sensors go to sensor models
      | 2. To_plants: Signals that are not actually sensed by sensors but are utilized by the rest of the plant and actually happen physically
      | Component_Logging: Logs both the signal kinds before going through sensor
  note: Motor Speed
  From_Actuators : Inport
  Sensor_Feedback : Inport  Port=2
  BAS Max Torque Curve : Lookup  InputValues=Plants.BAS.Mdl.Plant.max_min_w  Table=Plants.BAS.Mdl.Plant.T_max_Peak  LookUpMeth=Interpolation-Use End Values  SaturateOnIntegerOverflow=on
  BAS Min Torque Curve : Lookup  InputValues=Plants.BAS.Mdl.Plant.max_min_w  Table=Plants.BAS.Mdl.Plant.T_min_Peak  LookUpMeth=Interpolation-Use End Values  SaturateOnIntegerOverflow=on
  Bus Selector : BusSelector  OutputSignals=BAS_Torque_Command_Nm
  Bus Selector1 : BusSelector  OutputSignals=BAS_Speed_rad_per_s
  Ideal Torque Source : fl_lib/Mechanical/Mechanical Sources/Ideal Torque Source
  Inertia : fl_lib/Mechanical/Rotational Elements/Inertia  inertia=0.02 kg*m^2  w_specify=off  w_priority=High  w=0 rad/s  t_specify=off  t_priority=High  t=0 N*m
  Mechanical Rotational Reference : fl_lib/Mechanical/Rotational Elements/Mechanical Rotational Reference
  Saturation Dynamic1 : simulink/Discontinuities/Saturation Dynamic  OutMin=[]  OutMax=[]  OutDataTypeStr=Inherit: Same as second input  OutDataType=sfix(16)  OutScaling=2^-10  DoSatur=off
  Simulink-PS Converter : nesl_utility/Simulink-PS Converter  PhysicalDomain=network_engine_domain  SubClassName=ps_input  LeftPortType=input  RightPortType=output  PseudoPeriodic=off  Frequencies=[]  NoiseDistribution=none  NoiseParameters=[]  Unit=N*m  AffineConversion=off  InputFiltering=off  SimscapeFilterOrder=1  InputFilterTimeConstant=0.001  UdotUserProvided=1
  To_Sensors : PMIOPort  Port=1  Side=Right
  wires:
  From_Actuators/1 -> Bus Selector/1
  BAS Max Torque Curve/1 -> Saturation Dynamic1/1
  BAS Min Torque Curve/1 -> Saturation Dynamic1/3
  Saturation Dynamic1/1 -> Simulink-PS Converter/1  "BAS_Torque_Out_Nm"
  Bus Selector1/1 -> BAS Min Torque Curve/1, BAS Max Torque Curve/1  "<BAS_Speed_rad_per_s>"
  Sensor_Feedback/1 -> Bus Selector1/1
  Bus Selector/1 -> Saturation Dynamic1/2  "<BAS_Torque_Command_Nm>"
  connections:
  Mechanical Rotational Reference/LConn1 -- Ideal Torque Source/RConn2
  Ideal Torque Source/RConn1 -- Simulink-PS Converter/RConn1
  Ideal Torque Source/LConn1 -- Inertia/LConn1 -- To_Sensors/RConn1

== system EcoSIM3_P2_C2_WIP/Powertrain/BAS Motor/ Compnent Model/Sensors ==
  note: Sensor Model: Place where we add Corrupter
  Bus Creator : BusCreator  Inputs=3
  Ideal Rotational Motion Sensor : fl_lib/Mechanical/Mechanical Sensors/Ideal Rotational Motion Sensor  offset=0 rad
  Ideal Torque Sensor : fl_lib/Mechanical/Mechanical Sensors/Ideal Torque Sensor
  Mechanical Rotational Reference1 : fl_lib/Mechanical/Rotational Elements/Mechanical Rotational Reference
  PS-Simulink Converter : nesl_utility/PS-Simulink Converter  PhysicalDomain=network_engine_domain  SubClassName=ps_output  LeftPortType=input  RightPortType=output  PseudoPeriodic=off  Frequencies=[]  Unit=rad/s  AffineConversion=off
  PS-Simulink Converter1 : nesl_utility/PS-Simulink Converter  PhysicalDomain=network_engine_domain  SubClassName=ps_output  LeftPortType=input  RightPortType=output  PseudoPeriodic=off  Frequencies=[]  Unit=N*m  AffineConversion=off
  Product : Product
  Sensor lag : Subsystem
  Sensor lag1 : Subsystem
  Shaft : PMIOPort  Port=1  Side=Left
  To_Belt : PMIOPort  Port=2  Side=Right
  Sensor Out : Outport
  Battery : Outport  Port=2
  wires:
  Bus Creator/1 -> Sensor Out/1  "BAS_Sensor_Out"
  Sensor lag/1(o) -> Product/1, Bus Creator/1  "BAS_Speed_rad_per_s"
  PS-Simulink Converter1/1 -> Sensor lag1/1(i)  "BAS_Torque_Out_Nm"
  Product/1 -> Battery/1, Bus Creator/3  "BAS_Power_Out_W"
  PS-Simulink Converter/1 -> Sensor lag/1(i)  "BAS_Speed_rad_per_s"
  Sensor lag1/1(o) -> Product/2, Bus Creator/2  "BAS_Torque_Out_Nm"
  connections:
  Shaft/RConn1 -- Ideal Rotational Motion Sensor/LConn1 -- Ideal Torque Sensor/LConn1
  Ideal Rotational Motion Sensor/RConn1 -- Mechanical Rotational Reference1/LConn1
  PS-Simulink Converter1/LConn1 -- Ideal Torque Sensor/RConn2
  PS-Simulink Converter/LConn1 -- Ideal Rotational Motion Sensor/RConn2
  To_Belt/RConn1 -- Ideal Torque Sensor/RConn1

== system EcoSIM3_P2_C2_WIP/Powertrain/BAS Motor/Soft ECU/Algorithm ==
  note: Inputs:
      | BAS Speed
      | BAS Torque
      | ModeReq
      | IQ_Limit
      | IQ_Command
      | BAS_Powerup
  note: Sensor signals getting transmitted over CAN are selected here
  note: Notes:
      | 1. Mode Request is similar to Inverter Enable / Disable (to be received from the supervisory controller)
      | 2. Motor Fault is detected by a fault appearing at any of the phases of the motor (other faults can be incorporated in the Fault Subsystem)
  Inputs : Inport
  BAS Stateflow : Stateflow chart  TreatAsAtomicUnit=on
  Bus Creator : BusCreator  Inputs=8
  Bus Selector : BusSelector  OutputSignals=Fault_U,Fault_V,Fault_W
  Bus Selector1 : BusSelector  OutputSignals=BAS_Sensor_Out.BAS_Torque_Out_Nm,BAS_Sensor_Out.BAS_Speed_rad_per_s,BAS_SoftECU_Receive.BAS_Electrical.BAS_Powerup,BAS_SoftECU_Receive.BAS_CAN.SetValues.ModeReq,BAS_Sensor_Out.BAS_Speed_rad_per_s,BAS_SoftECU_Receive.BAS_CAN.SetValues.IQ_Command
  Bus Selector2 : BusSelector  OutputSignals=Motor_MaxSpeed,POST_Fault
  Constant : Constant  Value=Plants.Belt.GR  SampleTime=0.01
  Contactor_Status : Constant
  EEPROM Parameters : Subsystem
  Faults : Subsystem
  Logical Operator : Logic  AllPortsSameDT=off  OutDataTypeStr=boolean
  Scope : Scope
      settings: SaveName=ScopeData43
  Torque Determination : Subsystem
  Outputs : Outport
  wires:
  Bus Selector1/1 -> Bus Creator/1  "<BAS_Torque_Out_Nm>"
  Constant/1 -> BAS Stateflow/7(BeltRatio)
  Bus Selector1/5 -> Torque Determination/1(Speed)  "<BAS_Speed_rad_per_s>"
  Bus Selector1/2 -> Scope/1, BAS Stateflow/1(MotorSpeed), Bus Creator/2  "<BAS_Speed_rad_per_s>"
  Bus Selector1/6 -> Torque Determination/2(IQ)  "<IQ_Command>"
  Torque Determination/1(Out1) -> BAS Stateflow/4(Torque_Command)
  Bus Selector2/1 -> BAS Stateflow/5(MotorMaxSpeed)  "<Motor_MaxSpeed>"
  Bus Selector2/2 -> BAS Stateflow/6(POST_Fault)  "<POST_Fault>"
  Faults/1(MotorFault) -> BAS Stateflow/8(MotorFault)
  Bus Selector1/4 -> BAS Stateflow/3(ModeRequest)  "<ModeReq>"
  Bus Selector1/3 -> Logical Operator/1  "<BAS_Powerup>"
  Inputs/1 -> Bus Selector1/1
  BAS Stateflow/3(FaultState) -> Bus Creator/5  "BAS_Fault_Status"
  Bus Selector/1 -> Bus Creator/6  "<Fault_U>"
  Bus Selector/2 -> Bus Creator/7  "<Fault_V>"
  Bus Selector/3 -> Bus Creator/8  "<Fault_W>"
  Faults/2(CAN) -> Bus Selector/1
  Bus Creator/1 -> Outputs/1  "BAS_CAN_Out"
  BAS Stateflow/2(InverterStatusMode) -> Bus Creator/4  "BAS_Status_Mode"
  BAS Stateflow/1(Commanded_Torque) -> Bus Creator/3  "BAS_Torque_Command_Nm"
  Logical Operator/1 -> BAS Stateflow/2(Power_up)  "Power_up"
  Contactor_Status/1 -> Logical Operator/2  "batt_mainc_stat"
  EEPROM Parameters/1(EEPROM param) -> Bus Selector2/1

== system EcoSIM3_P2_C2_WIP/Powertrain/BAS Motor/Soft ECU/Inputs ==
  note: Do the input conditioning (if any) required by the
      | Algorith
  note: Select the CAN signals
  note: Combine all the Signals that go to the
      | Soft ECU Algorithm:
      | -Calculated Signals from Sensors and CAN
      | -Signalfrom sensors pass through because they
      | need to be sent out over the CAN by the ECU
  CAN_In : Inport
  Sensors : Inport  Port=2
  Bus Creator : BusCreator  Inputs=2
  To_Algorithm : Outport
  wires:
  Sensors/1 -> Bus Creator/1
  Bus Creator/1 -> To_Algorithm/1  "Component_to_Alg"
  CAN_In/1 -> Bus Creator/2

== system EcoSIM3_P2_C2_WIP/Powertrain/BAS Motor/Soft ECU/Inputs1 ==
  From Algorithm : Inport
  Bus Creator1 : BusCreator  Inputs=2
  Bus Creator3 : BusCreator  Inputs=8
  Bus Selector : BusSelector  OutputSignals=BAS_Speed_rad_per_s,BAS_Torque_Command_Nm,BAS_Status_Mode,BAS_Torque_Out_Nm,BAS_Fault_Status,Fault_U,Fault_V,Fault_W
  CAN Out : Outport
  Actuator Cmds : Outport  Port=2
  wires:
  From Algorithm/1 -> Bus Selector/1
  Bus Creator1/1 -> Actuator Cmds/1  "BAS_Actuator_Cmds"
  Bus Creator3/1 -> CAN Out/1  "BAS_CAN_Out"
  Bus Selector/1 -> Bus Creator3/1, Bus Creator1/1  "<BAS_Speed_rad_per_s>"
  Bus Selector/2 -> Bus Creator3/2, Bus Creator1/2  "<BAS_Torque_Command_Nm>"
  Bus Selector/3 -> Bus Creator3/3  "<BAS_Status_Mode>"
  Bus Selector/8 -> Bus Creator3/7  "<Fault_W>"
  Bus Selector/7 -> Bus Creator3/6  "<Fault_V>"
  Bus Selector/6 -> Bus Creator3/5  "<Fault_U>"
  Bus Selector/5 -> Bus Creator3/4  "<BAS_Fault_Status>"
  Bus Selector/4 -> Bus Creator3/8  "<BAS_Torque_Out_Nm>"

== system EcoSIM3_P2_C2_WIP/Powertrain/Charger/Soft ECU/Algorithm ==
  note: Both outputs are digital signals
  note: Signals like T& E are used to calculate whatever is required by Soft ECU
  Inputs : Inport
  Bus Creator1 : BusCreator  Inputs=3
  Bus Selector : BusSelector  OutputSignals=AC_Supply,PON
  Chart : Stateflow chart  TreatAsAtomicUnit=on
  Outputs : Outport
  tag scope: Charger_On=global
  wires:
  Bus Creator1/1 -> Outputs/1  "Brusa_SoftECU_Out"
  Inputs/1 -> Bus Selector/1
  Bus Selector/1 -> Chart/1(AC_Supply)  "<AC_Supply>"
  Bus Selector/2 -> Chart/2(PON)  "<PON>"
  Chart/1(chga_wake) -> Bus Creator1/1
  Chart/2(GCM_Wakeup_charge) -> Bus Creator1/2
  Chart/3(charge_start) -> [Charger_On], Bus Creator1/3

== system EcoSIM3_P2_C2_WIP/Powertrain/Charger/Soft ECU/Inputs ==
  note: Combine all the Signals that go to the
      | Soft ECU Algorithm:
      | -Calculated Signals from Sensors and CAN
      | -Signalfrom sensors pass through because they
      | need to be sent out over the CAN by the ECU
  note: Select the Sensor signals
  note: Select the CAN signals
  FromESS1 : Inport
  Supply : Inport  Port=2
  Bus Creator : BusCreator  Inputs=2
  To_Algorithm : Outport
  wires:
  Supply/1 -> Bus Creator/2  "AC_Supply"
  Bus Creator/1 -> To_Algorithm/1  "Inputs"
  FromESS1/1 -> Bus Creator/1

== system EcoSIM3_P2_C2_WIP/Powertrain/Charger/Soft ECU/Outputs ==
  note: Select the Sensor signals
  From Algorithm : Inport
  Bus Creator : BusCreator  Inputs=2
  Bus Creator1 : BusCreator  Inputs=1
  Bus Selector : BusSelector  OutputSignals=chga_wake,GCM_Wakeup_charge,charge_start
  ToECUs : Outport
  Actuator_Cmds : Outport  Port=2
  wires:
  From Algorithm/1 -> Bus Selector/1
  Bus Selector/1 -> Bus Creator/1  "<chga_wake>"
  Bus Selector/2 -> Bus Creator/2  "<GCM_Wakeup_charge>"
  Bus Creator/1 -> ToECUs/1  "Brusa_Out"
  Bus Selector/3 -> Bus Creator1/1  "<charge_start>"
  Bus Creator1/1 -> Actuator_Cmds/1  "Actuator_Cmds"

== system EcoSIM3_P2_C2_WIP/Powertrain/Clutch_Transmission1/CP1 SoftEcu/Algorithm ==
  note: Signals like T& E are used to calculate whatever is required by Soft ECU
  note: Sensor signals getting transmitted over CAN are selected here
  note: Sensor signals getting transmitted over CAN are bussed together here
  note: Cignals getting transmitted to Actuators are bussed together here
  Inputs : Inport
  Bus Creator : BusCreator  Inputs=2
  Bus Creator1 : BusCreator  Inputs=1
  Bus Creator2 : BusCreator  Inputs=1
  Bus Selector : BusSelector  OutputSignals=Clutch_Request,Sensor_Out.Clutch_Sensor_Out.Clutch_Pressure
  Chart : Stateflow chart  TreatAsAtomicUnit=on
  Memory : Memory  X0=120
  Outputs : Outport
  wires:
  Bus Creator/1 -> Outputs/1
  Memory/1 -> Chart/2(Clutch_Pressure)
  Bus Selector/1 -> Chart/1(Clutch_Request)  "<Clutch_Request>"
  Chart/2(Clutch_Sw) -> Bus Creator2/1  "Clutch_Sw"
  Bus Selector/2 -> Memory/1  "<Clutch_Pressure>"
  Bus Creator2/1 -> Bus Creator/2  "Clutch_CAN_Out"
  Bus Creator1/1 -> Bus Creator/1  "Component_Actuator_Commands"
  Chart/1(Clutch_Engage) -> Bus Creator1/1  "Clutch_Engage"
  Inputs/1 -> Bus Selector/1

== system EcoSIM3_P2_C2_WIP/Powertrain/Clutch_Transmission1/CP1 SoftEcu/Inputs ==
  note: Do the input conditioning (if any) required by the
      | Algorith
  note: Select the CAN signals
  note: Select the Sensor signals
  note: Combine all the Signals that go to the
      | Soft ECU Algorithm:
      | -Calculated Signals from Sensors and CAN
      | -Signalfrom sensors pass through because they
      | need to be sent out over the CAN by the ECU
  Sensors : Inport
  From GCM : Inport  Port=2
  Bus Creator : BusCreator  Inputs=2
  Bus Selector : BusSelector  OutputSignals=Clutch_Request
  To_Algorithm : Outport
  wires:
  Bus Selector/1 -> Bus Creator/2  "<Clutch_Request>"
  From GCM/1 -> Bus Selector/1
  Sensors/1 -> Bus Creator/1  "Sensor_Out"
  Bus Creator/1 -> To_Algorithm/1  "Component_to_Alg"

== system EcoSIM3_P2_C2_WIP/Powertrain/Clutch_Transmission1/CP1 SoftEcu/Inputs1 ==
  From Algorithm : Inport
  Bus Selector : BusSelector  OutputSignals=Component_Actuator_Commands.Clutch_Engage,Clutch_CAN_Out
  Actuator Cmd : Outport
  To GCM : Outport  Port=2
  wires:
  Bus Selector/2 -> To GCM/1  "<Clutch_CAN_Out>"
  Bus Selector/1 -> Actuator Cmd/1  "<Clutch_Engage>"
  From Algorithm/1 -> Bus Selector/1  "Sensor_Out"

== system EcoSIM3_P2_C2_WIP/Powertrain/Clutch_Transmission1/Clutch_Plant/Custom Clutch ==
  -1 : fl_lib/Physical Signals/Functions/PS Gain  gain=-1
  Dynamic friction coefficient lookup table : fl_lib/Physical Signals/Lookup Tables/PS Lookup Table (1D)  x_t=[ 0 0.1 0.2 0.3 0.4 0.5 1 2 5 10 100 1000 ]  y_t=[ 0.29 0.28 0.26 0.22 0.21 0.2 0.2 0.19 0.19 0.19 0.19 0.19 ]  interp_method=1  extrap_method=1
  Effective radius : fl_lib/Physical Signals/Functions/PS Gain  gain=0.3
  Fundamental Friction Clutch : sdl_lib/Clutches/Fundamental Components/Fundamental Friction Clutch  unidirectional=0  w_tol=0.001 rad/s  initial_state_locked=0
  PS Abs : fl_lib/Physical Signals/Nonlinear Operators/PS Abs
  PS Product1 : fl_lib/Physical Signals/Functions/PS Product
  PS-Simulink Converter1 : nesl_utility/PS-Simulink Converter  PhysicalDomain=network_engine_domain  SubClassName=ps_output  LeftPortType=input  RightPortType=output  PseudoPeriodic=off  Frequencies=[]  Unit=rad/s  AffineConversion=off
  Peak force : fl_lib/Physical Signals/Functions/PS Gain  gain=10
  Slip(rad/s) : Scope
      settings: YMin=-4  YMax=1
  Static/dynamic friction ratio : fl_lib/Physical Signals/Functions/PS Gain  gain=1.1
  "[0, inf]" : fl_lib/Physical Signals/Nonlinear Operators/PS Saturation  upper_limit=inf  lower_limit=0
  P : PMIOPort  Port=1  Side=Left
  Mode : PMIOPort  Port=2  Side=Right
  F : PMIOPort  Port=3  Side=Right
  B : PMIOPort  Port=4  Side=Left
  wires:
  PS-Simulink Converter1/1 -> Slip(rad/s)/1
  connections:
  PS Abs/RConn1 -- Dynamic friction coefficient lookup table/LConn1
  -1/RConn1 -- Fundamental Friction Clutch/LConn3
  Dynamic friction coefficient lookup table/RConn1 -- PS Product1/LConn2
  Static/dynamic friction ratio/LConn1 -- Fundamental Friction Clutch/LConn1 -- Effective radius/RConn1
  Static/dynamic friction ratio/RConn1 -- -1/LConn1 -- Fundamental Friction Clutch/LConn2
  P/RConn1 -- "[0, inf]"/LConn1
  B/RConn1 -- Fundamental Friction Clutch/LConn4
  PS Abs/LConn1 -- Fundamental Friction Clutch/RConn1 -- PS-Simulink Converter1/LConn1
  Fundamental Friction Clutch/RConn2 -- Mode/RConn1
  Fundamental Friction Clutch/RConn3 -- F/RConn1
  "[0, inf]"/RConn1 -- Peak force/LConn1
  PS Product1/RConn1 -- Effective radius/LConn1
  Peak force/RConn1 -- PS Product1/LConn1

== system EcoSIM3_P2_C2_WIP/Powertrain/Clutch_Transmission1/Clutch_Plant/Sensors ==
  Clutch_Pressure : Inport
  Bus Creator : BusCreator  Inputs=1
  Ideal Rotational Motion Sensor : fl_lib/Mechanical/Mechanical Sensors/Ideal Rotational Motion Sensor  offset=0 rad
  Ideal Torque Sensor : fl_lib/Mechanical/Mechanical Sensors/Ideal Torque Sensor
  Mechanical Rotational Reference1 : fl_lib/Mechanical/Rotational Elements/Mechanical Rotational Reference
  PS-Simulink Converter : nesl_utility/PS-Simulink Converter  PhysicalDomain=network_engine_domain  SubClassName=ps_output  LeftPortType=input  RightPortType=output  PseudoPeriodic=off  Frequencies=[]  Unit=rad/s  AffineConversion=off
  PS-Simulink Converter1 : nesl_utility/PS-Simulink Converter  PhysicalDomain=network_engine_domain  SubClassName=ps_output  LeftPortType=input  RightPortType=output  PseudoPeriodic=off  Frequencies=[]  Unit=N*m  AffineConversion=off
  Terminator : Terminator
  Terminator1 : Terminator
  Shaft : PMIOPort  Port=1  Side=Left
  To_Trans : PMIOPort  Tag=PMCPort  Port=2  Side=Right
  Clutch_Status : Outport
  wires:
  Bus Creator/1 -> Clutch_Status/1  "Clutch_Sensor_Out"
  Clutch_Pressure/1 -> Bus Creator/1  "Clutch_Pressure"
  PS-Simulink Converter1/1 -> Terminator1/1  "Clutch_Torque_Out_Nm"
  PS-Simulink Converter/1 -> Terminator/1  "Clutch_Speed_rad_per_s"
  connections:
  To_Trans/RConn1 -- Ideal Torque Sensor/RConn1
  PS-Simulink Converter1/LConn1 -- Ideal Torque Sensor/RConn2
  PS-Simulink Converter/LConn1 -- Ideal Rotational Motion Sensor/RConn2
  Ideal Rotational Motion Sensor/RConn1 -- Mechanical Rotational Reference1/LConn1
  Ideal Rotational Motion Sensor/LConn1 -- Shaft/RConn1 -- Ideal Torque Sensor/LConn1

== system EcoSIM3_P2_C2_WIP/Powertrain/Clutch_Transmission1/GCM/GCM Soft ECU ==
  Inputs : Inport
  Bus Creator : BusCreator
  Bus Selector : BusSelector  OutputSignals=Trans_Receive.Gear_Request,SoftECU_Out.Trans_CAN_Out.Actual_Gear
  Display : Display
  Display1 : Display
  Memory : Memory
  Shift Signal Generator : Stateflow chart  TreatAsAtomicUnit=on
  Outputs : Outport
  wires:
  Memory/1 -> Shift Signal Generator/2(Actual_Gear), Bus Creator/4, Display1/1  "Actual_Gear"
  Bus Creator/1 -> Outputs/1
  Bus Selector/2 -> Memory/1  "<Actual_Gear>"
  Bus Selector/1 -> Shift Signal Generator/1(Gear_Request), Display/1  "<Gear_Request>"
  Shift Signal Generator/3(Downshift_Sw) -> Bus Creator/3  "Downshift_Sw"
  Shift Signal Generator/2(Upshift_Sw) -> Bus Creator/2  "Upshift_Sw"
  Inputs/1 -> Bus Selector/1
  Shift Signal Generator/1(Clutch_Request) -> Bus Creator/1  "Clutch_Request"

== system EcoSIM3_P2_C2_WIP/Powertrain/Clutch_Transmission1/GCM/Inputs ==
  note: Combine all the Signals that go to the
      | Soft ECU Algorithm:
      | -Calculated Signals from Sensors and CAN
      | -Signalfrom sensors pass through because they
      | need to be sent out over the CAN by the ECU
  note: Select the Sensor signals
  note: Select the CAN signals
  note: Do the input conditioning (if any) required by the
      | Algorith
  From SoftECU : Inport
  CAN_In : Inport  Port=2
  Bus Creator : BusCreator  Inputs=2
  Bus Selector : BusSelector  OutputSignals=Clutch_Trans_SoftECU_Receive.Clutch_Trans_CAN.Trans_Receive
  To_Algorithm : Outport
  wires:
  Bus Selector/1 -> Bus Creator/2  "<Trans_Receive>"
  Bus Creator/1 -> To_Algorithm/1  "Component_to_Alg"
  From SoftECU/1 -> Bus Creator/1
  CAN_In/1 -> Bus Selector/1

== system EcoSIM3_P2_C2_WIP/Powertrain/Clutch_Transmission1/GCM/Outputs ==
  From Algorithm : Inport
  Bus Creator : BusCreator  Inputs=3
  Bus Creator1 : BusCreator  Inputs=1
  Bus Selector : BusSelector  OutputSignals=Actual_Gear,Clutch_Request,Upshift_Sw,Downshift_Sw
  CAN_Out : Outport
  To_SoftECU : Outport  Port=2
  wires:
  Bus Selector/1 -> Bus Creator1/1  "<Actual_Gear>"
  Bus Creator1/1 -> CAN_Out/1  "Message_1"
  Bus Creator/1 -> To_SoftECU/1  "SoftECU_Receive"
  Bus Selector/4 -> Bus Creator/3  "<Downshift_Sw>"
  Bus Selector/3 -> Bus Creator/2  "<Upshift_Sw>"
  Bus Selector/2 -> Bus Creator/1  "<Clutch_Request>"
  From Algorithm/1 -> Bus Selector/1  "Sensor_Out"
